simulink model "control__effort"  (R2020a)
settings: Solver=VariableStepAuto  StartTime=0.0  StopTime=10.0  RelTol=1e-3
libraries: simulink x1
settings Model: Creator=Iman  LastModifiedBy=Iman

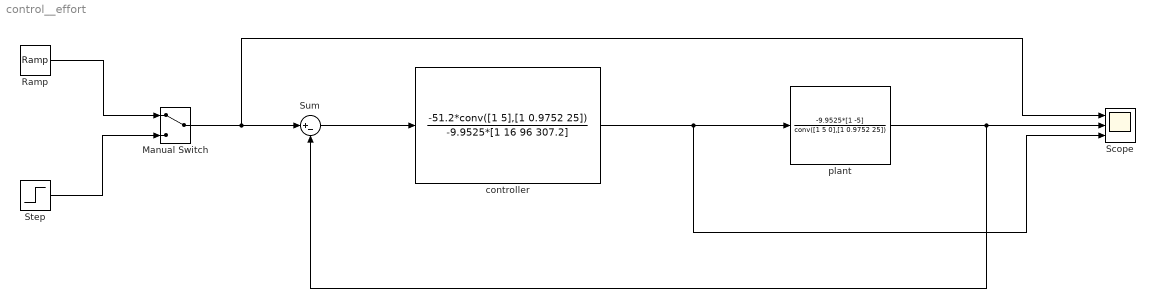
== system control__effort ==
  Manual Switch : ManualSwitch
  Ramp : simulink/Sources/Ramp  slope=1  start=0  InitialOutput=0
  Scope : Scope  NumInputPorts=3
  Step : Step  Time=0  SampleTime=0
  Sum : Sum  Inputs=|+-
  controller : TransferFcn  Numerator=-51.2*conv([1 5],[1 0.9752 25])  Denominator=-9.9525*[1 16 96 307.2]
  "plant " : TransferFcn  Numerator=-9.9525*[1 -5]  Denominator=conv([1 5 0],[1 0.9752 25])
  wires:
  Step/1 -> Manual Switch/2
  Ramp/1 -> Manual Switch/1
  Sum/1 -> controller/1
  "plant "/1 -> Sum/2, Scope/2
  Manual Switch/1 -> Scope/1, Sum/1
  controller/1 -> Scope/3, "plant "/1
